simulink model "Stamp_tunet_vs_ikketunet"  (R2022a)
settings: Solver=VariableStepAuto  StartTime=0.0  StopTime=15  RelTol=1e-3
values from neighbouring files (symbols this model uses):
  B_s_f = 0.002833197    [Modell_verdier.m]
  B_s_t = 0.000183411    [Modell_verdier.m]
  C_D = 1.28    [Modell_verdier.m]
  Fb = 226    [Modell_verdier.m]
  g = 9.81    [Modell_verdier.m]
  I_stamp = 1.29837    [Modell_verdier.m]
  r_Fb = 0.036    [Modell_verdier.m]
  r_motor_stamp = 0.269    [Modell_verdier.m]
  tetthet_vann = 1000    [Modell_verdier.m]
  theta_motor_stamp = deg2rad(90-60.8)    [Modell_verdier.m]
libraries: simulink_extras x6, spsFirstOrderFilterLib x2
settings Model: Creator=andre  LastModifiedBy=andre

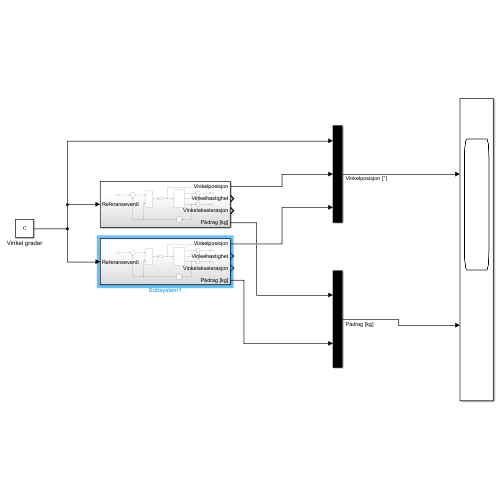
[thumbnail: Simulink's stored preview of the top-level diagram]
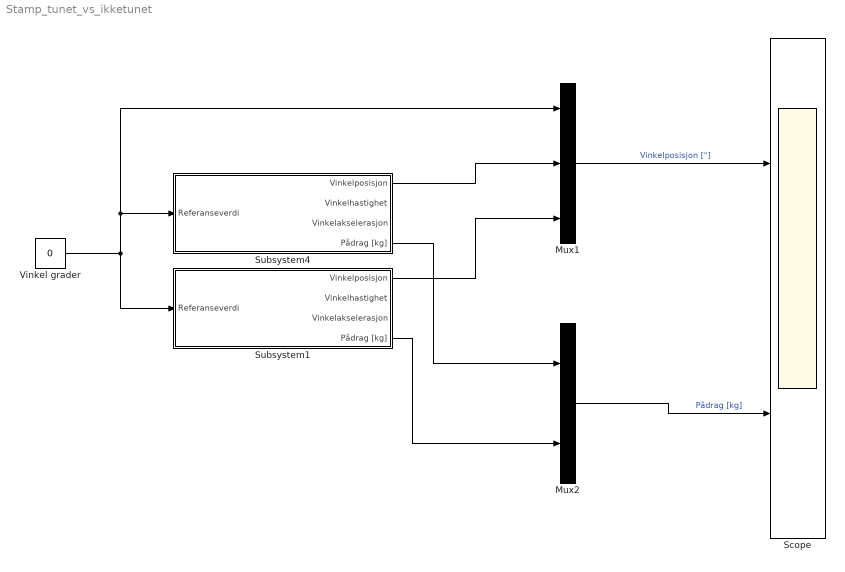
== system Stamp_tunet_vs_ikketunet ==
  Mux1 : Mux  Inputs=3
  Mux2 : Mux  Inputs=2
  Scope : Scope  NumInputPorts=2
  Subsystem1 : Subsystem
  Subsystem4 : Subsystem
  Vinkel grader : Constant  Value=0
  wires:
  Vinkel grader/1 -> Mux1/1, Subsystem4/1(Referanseverdi), Subsystem1/1(Referanseverdi)
  Subsystem4/1(Vinkelposisjon) -> Mux1/2
  Subsystem1/1(Vinkelposisjon) -> Mux1/3
  Subsystem4/4(Pådrag [kg]) -> Mux2/1
  Subsystem1/4(Pådrag [kg]) -> Mux2/2
  Mux1/1 -> Scope/1  "Vinkelposisjon [°]"
  Mux2/1 -> Scope/2  "Pådrag [kg]"

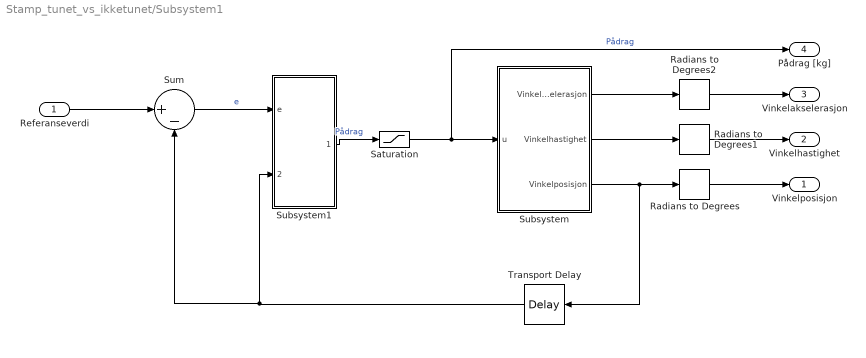
== system Stamp_tunet_vs_ikketunet/Subsystem1 ==
  Referanseverdi : Inport
  Radians to Degrees : simulink_extras/Transformations/Radians to Degrees
  Radians to Degrees1 : simulink_extras/Transformations/Radians to Degrees
  Radians to Degrees2 : simulink_extras/Transformations/Radians to Degrees
  Saturation : Saturate  UpperLimit=0.6  LowerLimit=-0.6
  Subsystem : Subsystem
  Subsystem1 : Subsystem
  Sum : Sum  Inputs=|+-
  Transport Delay : TransportDelay  DelayTime=0.2
  Vinkelposisjon : Outport
  Vinkelhastighet : Outport  Port=2
  Vinkelakselerasjon : Outport  Port=3
  Pådrag [kg] : Outport  Port=4
  wires:
  Saturation/1 -> Pådrag [kg]/1, Subsystem/1(u)  "Pådrag"
  Radians to Degrees1/1 -> Vinkelhastighet/1
  Subsystem/3(Vinkelposisjon) -> Transport Delay/1, Radians to Degrees/1
  Radians to Degrees/1 -> Vinkelposisjon/1
  Transport Delay/1 -> Sum/2, Subsystem1/2(y_sensor)
  Subsystem/1(" Vinkelakselerasjon") -> Radians to Degrees2/1
  Subsystem/2(" Vinkelhastighet") -> Radians to Degrees1/1
  Subsystem1/1(Pådrag) -> Saturation/1  "Pådrag"
  Sum/1 -> Subsystem1/1(e)  "e"
  Referanseverdi/1 -> Sum/1
  Radians to Degrees2/1 -> Vinkelakselerasjon/1

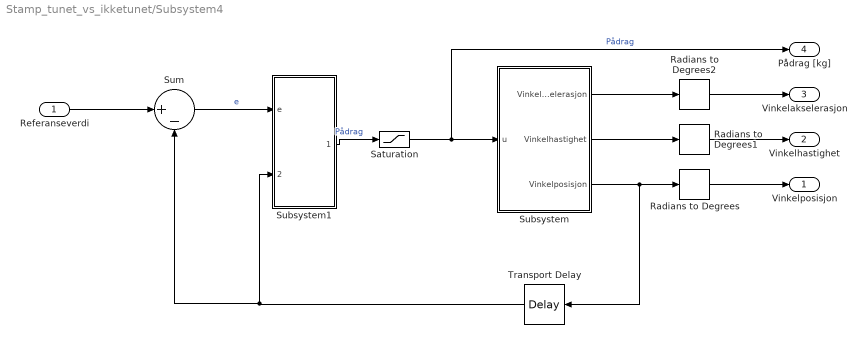
== system Stamp_tunet_vs_ikketunet/Subsystem4 ==
  Referanseverdi : Inport
  Radians to Degrees : simulink_extras/Transformations/Radians to Degrees
  Radians to Degrees1 : simulink_extras/Transformations/Radians to Degrees
  Radians to Degrees2 : simulink_extras/Transformations/Radians to Degrees
  Saturation : Saturate  UpperLimit=0.6  LowerLimit=-0.6
  Subsystem : Subsystem
  Subsystem1 : Subsystem
  Sum : Sum  Inputs=|+-
  Transport Delay : TransportDelay  DelayTime=0.2
  Vinkelposisjon : Outport
  Vinkelhastighet : Outport  Port=2
  Vinkelakselerasjon : Outport  Port=3
  Pådrag [kg] : Outport  Port=4
  wires:
  Saturation/1 -> Pådrag [kg]/1, Subsystem/1(u)  "Pådrag"
  Radians to Degrees1/1 -> Vinkelhastighet/1
  Subsystem/3(Vinkelposisjon) -> Transport Delay/1, Radians to Degrees/1
  Radians to Degrees/1 -> Vinkelposisjon/1
  Transport Delay/1 -> Sum/2, Subsystem1/2(y_sensor)
  Subsystem/1(" Vinkelakselerasjon") -> Radians to Degrees2/1
  Subsystem/2(" Vinkelhastighet") -> Radians to Degrees1/1
  Subsystem1/1(Pådrag) -> Saturation/1  "Pådrag"
  Sum/1 -> Subsystem1/1(e)  "e"
  Referanseverdi/1 -> Sum/1
  Radians to Degrees2/1 -> Vinkelakselerasjon/1

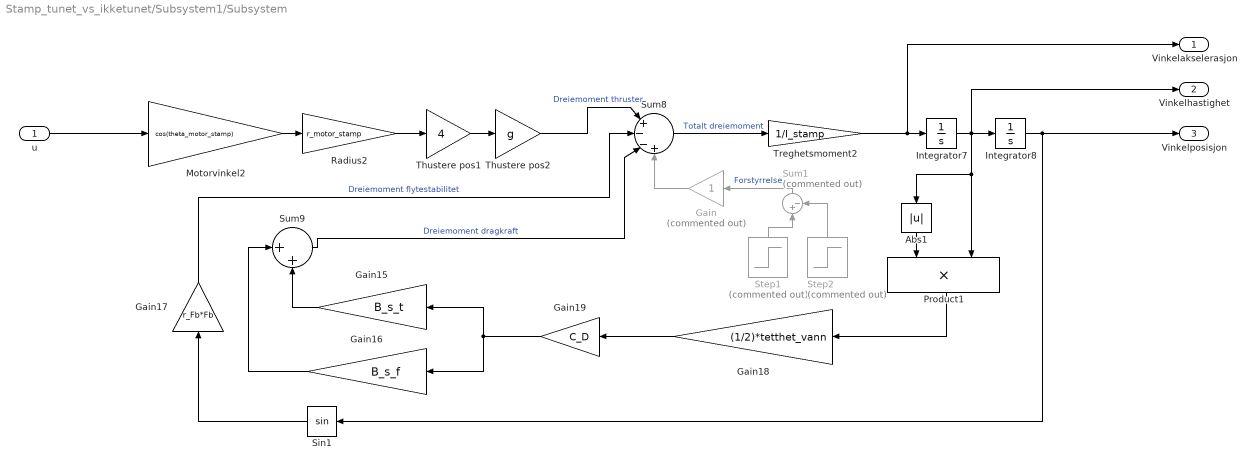
== system Stamp_tunet_vs_ikketunet/Subsystem1/Subsystem ==
  u : Inport
  Abs1 : Abs  SaturateOnIntegerOverflow=off
  Gain : Gain  Commented=on
  Gain15 : Gain  Gain=B_s_t
  Gain16 : Gain  Gain=B_s_f
  Gain17 : Gain  Gain=r_Fb*Fb
  Gain18 : Gain  Gain=(1/2)*tetthet_vann
  Gain19 : Gain  Gain=C_D
  Integrator7 : Integrator
  Integrator8 : Integrator  InitialCondition=2*pi/9
  Motorvinkel2 : Gain  Gain=cos(theta_motor_stamp)
  Product1 : Product
  Radius2 : Gain  Gain=r_motor_stamp
  Sin1 : Trigonometry
  Step1 : Step  Commented=on  Time=7  After=3.5  SampleTime=0
  Step2 : Step  Commented=on  Time=10  After=3.5  SampleTime=0
  Sum1 : Sum  Commented=on  Inputs=|+-
  Sum8 : Sum  Inputs=|+--+
  Sum9 : Sum  Inputs=|++
  Thustere pos1 : Gain  Gain=4
  Thustere pos2 : Gain  Gain=g
  Treghetsmoment2 : Gain  Gain=1/I_stamp
  " Vinkelakselerasjon" : Outport
  " Vinkelhastighet" : Outport  Port=2
  Vinkelposisjon : Outport  Port=3
  wires:
  Product1/1 -> Gain18/1
  Integrator8/1 -> Vinkelposisjon/1, Sin1/1
  Treghetsmoment2/1 -> " Vinkelakselerasjon"/1, Integrator7/1
  Thustere pos1/1 -> Thustere pos2/1
  Gain18/1 -> Gain19/1
  Thustere pos2/1 -> Sum8/1  "Dreiemoment thruster"
  Integrator7/1 -> " Vinkelhastighet"/1, Abs1/1, Product1/2, Integrator8/1
  Abs1/1 -> Product1/1
  Motorvinkel2/1 -> Radius2/1
  Gain19/1 -> Gain15/1, Gain16/1
  Gain17/1 -> Sum8/2  "Dreiemoment flytestabilitet"
  Gain16/1 -> Sum9/1
  Gain15/1 -> Sum9/2
  Radius2/1 -> Thustere pos1/1
  Sum9/1 -> Sum8/3  "Dreiemoment dragkraft"
  Sin1/1 -> Gain17/1
  Sum8/1 -> Treghetsmoment2/1  "Totalt dreiemoment"
  u/1 -> Motorvinkel2/1
  Step2/1 -> Sum1/2
  Gain/1 -> Sum8/4
  Sum1/1 -> Gain/1  "Forstyrrelse"
  Step1/1 -> Sum1/1

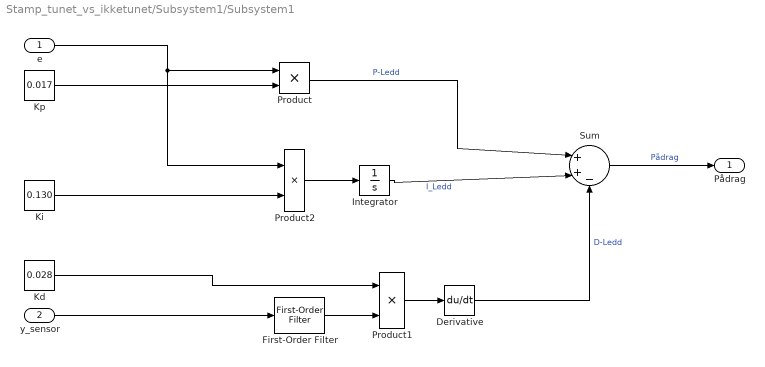
== system Stamp_tunet_vs_ikketunet/Subsystem1/Subsystem1 ==
  e : Inport
  y_sensor : Inport  Port=2
  Derivative : Derivative
  First-Order Filter : spsFirstOrderFilterLib/First-Order Filter  FilterType=Lowpass  Tc=(1.5/3.8)*0.05  Ts=0  Initialize=on  Vac_Init=[0, 0, 60]  Vdc_Init=0  PlotResponse=off  FreqRange="[0,  200,  1]"
  Integrator : Integrator  LimitOutput=on  UpperSaturationLimit=0.3  LowerSaturationLimit=-0.3
  Kd : Constant  Value=0.028
  Ki : Constant  Value=0.130
  Kp : Constant  Value=0.017
  Product : Product
  Product1 : Product
  Product2 : Product
  Sum : Sum  Inputs=|++-
  Pådrag : Outport
  wires:
  Product2/1 -> Integrator/1
  Kp/1 -> Product/2
  Product/1 -> Sum/1  "P-Ledd"
  y_sensor/1 -> First-Order Filter/1
  Kd/1 -> Product1/1
  e/1 -> Product/1, Product2/1
  Ki/1 -> Product2/2
  First-Order Filter/1 -> Product1/2
  Integrator/1 -> Sum/2  "I_Ledd"
  Sum/1 -> Pådrag/1  "Pådrag"
  Product1/1 -> Derivative/1
  Derivative/1 -> Sum/3  "D-Ledd"

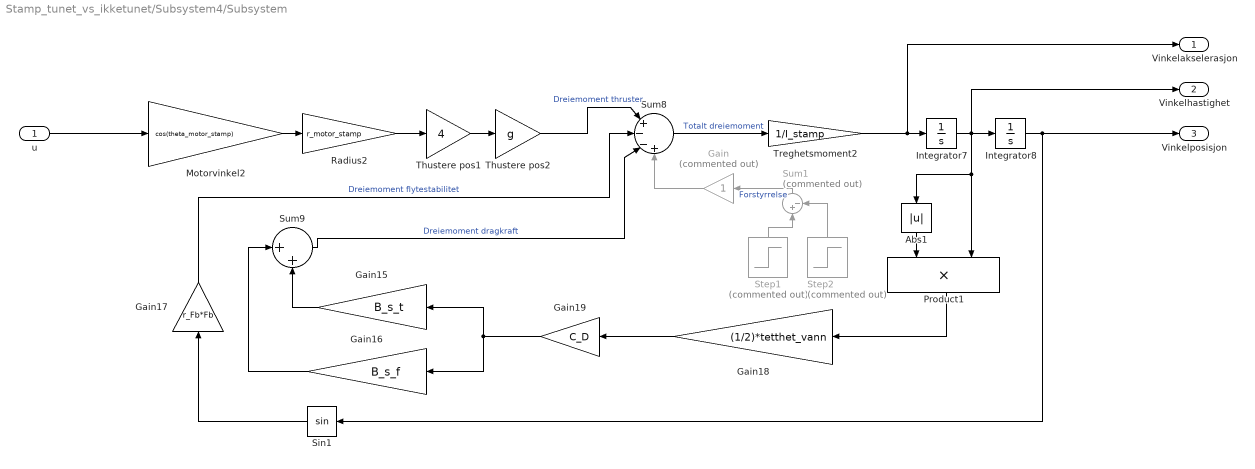
== system Stamp_tunet_vs_ikketunet/Subsystem4/Subsystem ==
  u : Inport
  Abs1 : Abs  SaturateOnIntegerOverflow=off
  Gain : Gain  Commented=on
  Gain15 : Gain  Gain=B_s_t
  Gain16 : Gain  Gain=B_s_f
  Gain17 : Gain  Gain=r_Fb*Fb
  Gain18 : Gain  Gain=(1/2)*tetthet_vann
  Gain19 : Gain  Gain=C_D
  Integrator7 : Integrator
  Integrator8 : Integrator  InitialCondition=2*pi/9
  Motorvinkel2 : Gain  Gain=cos(theta_motor_stamp)
  Product1 : Product
  Radius2 : Gain  Gain=r_motor_stamp
  Sin1 : Trigonometry
  Step1 : Step  Commented=on  Time=7  After=3.5  SampleTime=0
  Step2 : Step  Commented=on  Time=10  After=3.5  SampleTime=0
  Sum1 : Sum  Commented=on  Inputs=|+-
  Sum8 : Sum  Inputs=|+--+
  Sum9 : Sum  Inputs=|++
  Thustere pos1 : Gain  Gain=4
  Thustere pos2 : Gain  Gain=g
  Treghetsmoment2 : Gain  Gain=1/I_stamp
  " Vinkelakselerasjon" : Outport
  " Vinkelhastighet" : Outport  Port=2
  Vinkelposisjon : Outport  Port=3
  wires:
  Product1/1 -> Gain18/1
  Integrator8/1 -> Vinkelposisjon/1, Sin1/1
  Treghetsmoment2/1 -> " Vinkelakselerasjon"/1, Integrator7/1
  Thustere pos1/1 -> Thustere pos2/1
  Gain18/1 -> Gain19/1
  Thustere pos2/1 -> Sum8/1  "Dreiemoment thruster"
  Integrator7/1 -> " Vinkelhastighet"/1, Abs1/1, Product1/2, Integrator8/1
  Abs1/1 -> Product1/1
  Motorvinkel2/1 -> Radius2/1
  Gain19/1 -> Gain15/1, Gain16/1
  Gain17/1 -> Sum8/2  "Dreiemoment flytestabilitet"
  Gain16/1 -> Sum9/1
  Gain15/1 -> Sum9/2
  Radius2/1 -> Thustere pos1/1
  Sum9/1 -> Sum8/3  "Dreiemoment dragkraft"
  Sin1/1 -> Gain17/1
  Sum8/1 -> Treghetsmoment2/1  "Totalt dreiemoment"
  u/1 -> Motorvinkel2/1
  Step2/1 -> Sum1/2
  Gain/1 -> Sum8/4
  Sum1/1 -> Gain/1  "Forstyrrelse"
  Step1/1 -> Sum1/1

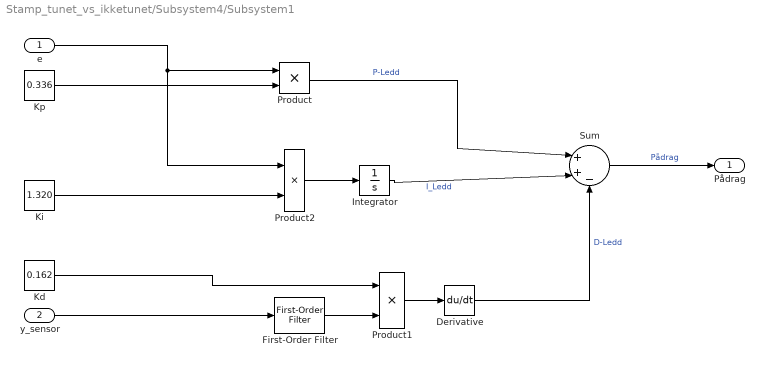
== system Stamp_tunet_vs_ikketunet/Subsystem4/Subsystem1 ==
  e : Inport
  y_sensor : Inport  Port=2
  Derivative : Derivative
  First-Order Filter : spsFirstOrderFilterLib/First-Order Filter  FilterType=Lowpass  Tc=(1.5/3.8)*0.05  Ts=0  Initialize=on  Vac_Init=[0, 0, 60]  Vdc_Init=0  PlotResponse=off  FreqRange="[0,  200,  1]"
  Integrator : Integrator  LimitOutput=on  UpperSaturationLimit=0.3  LowerSaturationLimit=-0.3
  Kd : Constant  Value=0.162
  Ki : Constant  Value=1.320
  Kp : Constant  Value=0.336
  Product : Product
  Product1 : Product
  Product2 : Product
  Sum : Sum  Inputs=|++-
  Pådrag : Outport
  wires:
  Product2/1 -> Integrator/1
  Kp/1 -> Product/2
  Product/1 -> Sum/1  "P-Ledd"
  y_sensor/1 -> First-Order Filter/1
  Kd/1 -> Product1/1
  e/1 -> Product/1, Product2/1
  Ki/1 -> Product2/2
  First-Order Filter/1 -> Product1/2
  Integrator/1 -> Sum/2  "I_Ledd"
  Sum/1 -> Pådrag/1  "Pådrag"
  Product1/1 -> Derivative/1
  Derivative/1 -> Sum/3  "D-Ledd"
